simulink model "center_out_3Dv2_ard2"  (Simulink 8.7)
settings: Solver=FixedStepDiscrete  StartTime=0.0  StopTime=Inf  FixedStep=.001  RelTol=1e-3
libraries: slrtlib x6, xpcnilib x5, dspsigops x2, limblab x2, IntelSMIlibR2007b x1, xpcobsoletelib x1, xpcrtudplib x1
CloseFcn:
  | rtwprivate ssgencode ModelCloseRequest rwalk_multi_local_v1
settings Model: Creator=limblab  LastModifiedBy=limblab  ExtModeArmWhenConnect=off
settings SolverCC: EnableConcurrentExecution=on
settings DataIOCC: LimitDataPoints=off  SaveFormat=StructureWithTime  SignalLoggingSaveFormat=ModelDataLogs  SaveState=on  SignalLoggingName=sigsOut
settings OptimizationCC: BlockReduction=off  BooleanDataType=off  OptimizeBlockIOStorage=off  BufferReuse=off  GlobalBufferReuse=off  ExpressionFolding=off  ExpressionDepthLimit=2147483647  LocalBlockOutputs=off  InitFltsAndDblsToZero=on
settings DebuggingCC: SaveWithParameterizedLinksMsg=none  SignalResolutionControl=TryResolveAllWithWarning  MultiTaskDSMMsg=warning  MultiTaskCondExecSysMsg=none  FcnCallInpInsideContextMsg=UseLocalSettings  StateNameClashWarn=warning
settings HardwareCC: ProdIntDivRoundTo=Zero  ProdEndianess=LittleEndian  ProdLongLongMode=on  ProdHWDeviceType=Generic->32-bit x86 compatible  TargetHWDeviceType=32-bit Generic
settings SFSimCC: SimParseCustomCode=off
settings RTWCC: SystemTargetFile=slrt.tlc  TemplateMakefile=slrt_default_tmf  Description=Simulink Real-Time  GenerateReport=on  RTWCompilerOptimization=on
settings SimulinkRealTimeCC: TargetFcnLib=ansi_tfl_tmw.mat  GeneratePreprocessorConditionals=Disable all

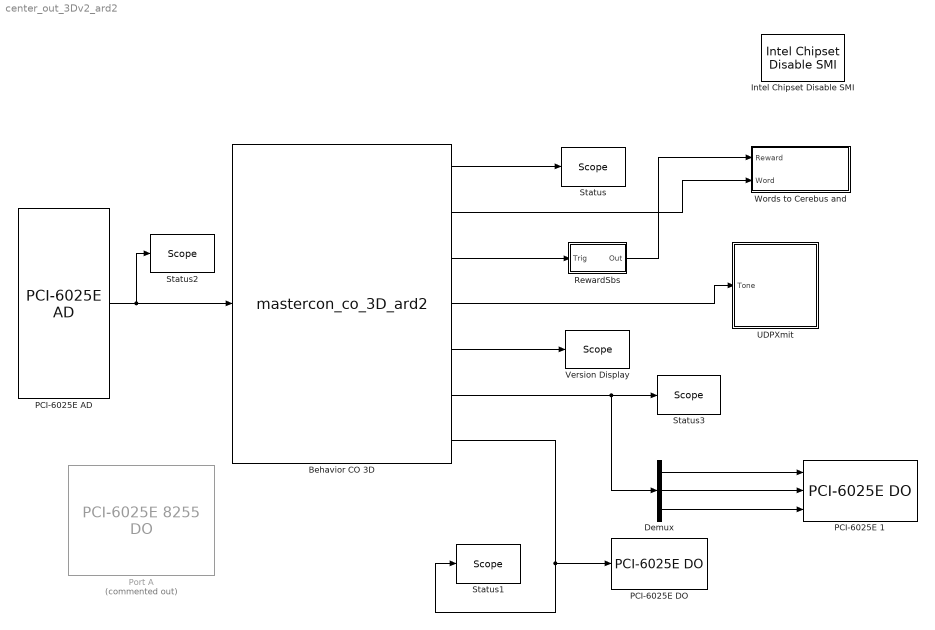
== system center_out_3Dv2_ard2 ==
  Behavior CO 3D : S-Function  FunctionName=mastercon_co_3D_ard2  Parameters=8 10 2.5 1 1 .5 1.5 .75 .25 1 1 10  SFunctionDeploymentMode=off  EnableBusSupport=off
      mask Display:
      | disp('Master Control')
      | port_label('input',1,'Target')
      | port_label('input',2,'Target 2')
      | port_label('output',1,'status')
      | port_label('output',2,'word')
      | port_label('output',3,'reward')
      | port_label('output',4,'tone')
      | port_label('output',5,'version')
      | port_label('output',6,'LEDs')
  Demux : Demux  Outputs=3
  Intel Chipset Disable SMI : IntelSMIlibR2007b/Intel Chipset Disable SMI
  PCI-6025E 1 : xpcnilib/Digital Output/E Series/PCI-6025E DO  channel=[3,7,6]  reset=[0]  initValue=[0]  sampletime=.001  slot=-1
  PCI-6025E AD : xpcnilib/A//D/E Series/PCI-6025E AD  channel=[7]  range=[-10]  coupling=[0]  sampletime=0.001  slot=-1
  PCI-6025E DO : xpcnilib/Digital Output/E Series/PCI-6025E DO  channel=[5]  reset=[1]  initValue=[0]  sampletime=0.001  slot=-1
  Port A : xpcnilib/Digital Output/E Series/PCI-6025E 8255 DO  Commented=on  channel=1:8  port=A  reset=[1]  initValue=[0]  chip=1  sampletime=-1  slot=-1
  RewardSbs : Subsystem
  Status : slrtlib/Displays and Logging/Scope   scopeno=1  scopetype=Target  autostart=on  viewmode=Numerical  formatstr='%6.0f state,%6.0f rewards,%6.0f aborts,%6.0f fails,%6.0f incompl'  grid=on  ylimits=[-10,10]  nosamples=10  noprepostsamples=0  interleave=10  triggermode=FreeRun  triggersignal=1  trigsignalfromport=off  triggerlevel=0.0  triggerslope=Either  triggerscope=1  triggersample=0  filename=data.dat  mode=Lazy  writesize=512  autorestart=off  dynamicfilemode=off  maxwritefilesize=512*1024^2
  Status1 : slrtlib/Displays and Logging/Scope   scopeno=3  scopetype=Target  autostart=on  viewmode=Numerical  formatstr='%1.0f IMU reset'  grid=on  ylimits=[-10,10]  nosamples=10  noprepostsamples=0  interleave=10  triggermode=FreeRun  triggersignal=1  trigsignalfromport=off  triggerlevel=0.0  triggerslope=Either  triggerscope=1  triggersample=0  filename=data.dat  mode=Lazy  writesize=512  autorestart=off  dynamicfilemode=off  maxwritefilesize=512*1024^2
  Status2 : slrtlib/Displays and Logging/Scope   scopeno=4  scopetype=Target  autostart=on  viewmode=Numerical  formatstr='%f Target1'  grid=on  ylimits=[-10,10]  nosamples=10  noprepostsamples=0  interleave=10  triggermode=FreeRun  triggersignal=1  trigsignalfromport=off  triggerlevel=0.0  triggerslope=Either  triggerscope=1  triggersample=0  filename=data.dat  mode=Lazy  writesize=512  autorestart=off  dynamicfilemode=off  maxwritefilesize=512*1024^2
  Status3 : slrtlib/Displays and Logging/Scope   scopeno=5  scopetype=Target  autostart=on  viewmode=Numerical  formatstr='%1.0f Out1,%1.0f Out2,%1.0f Out3'  grid=on  ylimits=[-10,10]  nosamples=10  noprepostsamples=0  interleave=10  triggermode=FreeRun  triggersignal=1  trigsignalfromport=off  triggerlevel=0.0  triggerslope=Either  triggerscope=1  triggersample=0  filename=data.dat  mode=Lazy  writesize=512  autorestart=off  dynamicfilemode=off  maxwritefilesize=512*1024^2
  UDPXmit : Subsystem
  Version Display : slrtlib/Displays and Logging/Scope   scopeno=2  scopetype=Target  autostart=on  viewmode=Numerical  formatstr='%6.0f major,%6.0f minor,%6.0f revision,%6.0f build'  grid=on  ylimits=[-10,10]  nosamples=10  noprepostsamples=0  interleave=10  triggermode=FreeRun  triggersignal=1  trigsignalfromport=off  triggerlevel=0.0  triggerslope=Either  triggerscope=1  triggersample=0  filename=data.dat  mode=Lazy  writesize=512  autorestart=off  dynamicfilemode=off  maxwritefilesize=512*1024^2
  "Words to Cerebus and " : Subsystem
  wires:
  Behavior CO 3D/1 -> Status/1
  Behavior CO 3D/2 -> "Words to Cerebus and "/2(Word)
  Behavior CO 3D/4 -> UDPXmit/1(Tone)
  Behavior CO 3D/5 -> Version Display/1
  Demux/1 -> PCI-6025E 1/1
  Demux/2 -> PCI-6025E 1/2
  Demux/3 -> PCI-6025E 1/3
  Behavior CO 3D/3 -> RewardSbs/1(Trig)
  RewardSbs/1(Out) -> "Words to Cerebus and "/1(Reward)
  Behavior CO 3D/6 -> Demux/1, Status3/1
  PCI-6025E AD/1 -> Behavior CO 3D/1, Status2/1
  Behavior CO 3D/7 -> Status1/1, PCI-6025E DO/1

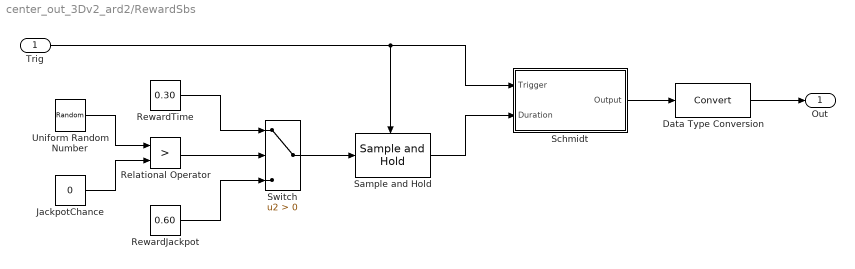
== system center_out_3Dv2_ard2/RewardSbs ==
  Trig : Inport
  Data Type Conversion : DataTypeConversion
  JackpotChance : Constant  Value=0
  Relational Operator : RelationalOperator  Operator=>  OutDataTypeStr=boolean
  RewardJackpot : Constant  Value=0.60
  RewardTime : Constant  Value=0.30
  Sample and Hold : dspsigops/Sample and Hold  trig=Rising edge  initCond=0  latchinput=off
  Schmidt : Subsystem
  Switch : Switch  Criteria=u2 > Threshold  ZeroCross=off
  Uniform Random Number : UniformRandomNumber  Minimum=0  Maximum=100  SampleTime=0.001
  Out : Outport
  wires:
  Trig/1 -> Schmidt/1(Trigger), Sample and Hold/Trigger
  Data Type Conversion/1 -> Out/1
  Schmidt/1(Output) -> Data Type Conversion/1
  Sample and Hold/1 -> Schmidt/2(Duration)
  RewardTime/1 -> Switch/1
  RewardJackpot/1 -> Switch/3
  Switch/1 -> Sample and Hold/1
  Uniform Random Number/1 -> Relational Operator/1
  Relational Operator/1 -> Switch/2
  JackpotChance/1 -> Relational Operator/2

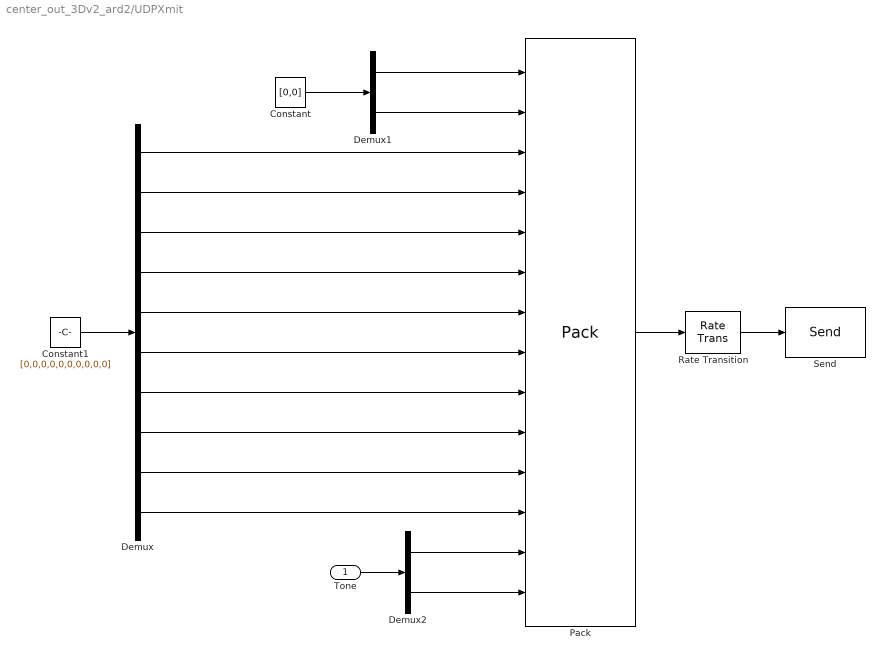
== system center_out_3Dv2_ard2/UDPXmit ==
  Tone : Inport
  Constant : Constant  Value=[0,0]
  Constant1 : Constant  Value=[0,0,0,0,0,0,0,0,0,0]
  Demux : Demux  Outputs=10
  Demux1 : Demux  Outputs=2
  Demux2 : Demux  Outputs=2
  Pack : xpcobsoletelib/Utilities/Pack   datatypes={'double', 'double','double','double','double','double','double','double','double','double','double','double','double','double'}  byteAlign=1
  Rate Transition : RateTransition
  Send : xpcrtudplib/Legacy UDP/Send   ipAddress=192.168.0.2  ipPort=25000  localPort=-1  vblLen=off  sampletime=.02
  wires:
  Rate Transition/1 -> Send/1
  Pack/1 -> Rate Transition/1
  Demux/10 -> Pack/12
  Demux/9 -> Pack/11
  Demux/8 -> Pack/10
  Demux/7 -> Pack/9
  Demux/6 -> Pack/8
  Demux/5 -> Pack/7
  Demux/4 -> Pack/6
  Demux/3 -> Pack/5
  Demux/2 -> Pack/4
  Demux/1 -> Pack/3
  Demux1/1 -> Pack/1
  Demux1/2 -> Pack/2
  Demux2/1 -> Pack/13
  Demux2/2 -> Pack/14
  Tone/1 -> Demux2/1
  Constant1/1 -> Demux/1
  Constant/1 -> Demux1/1

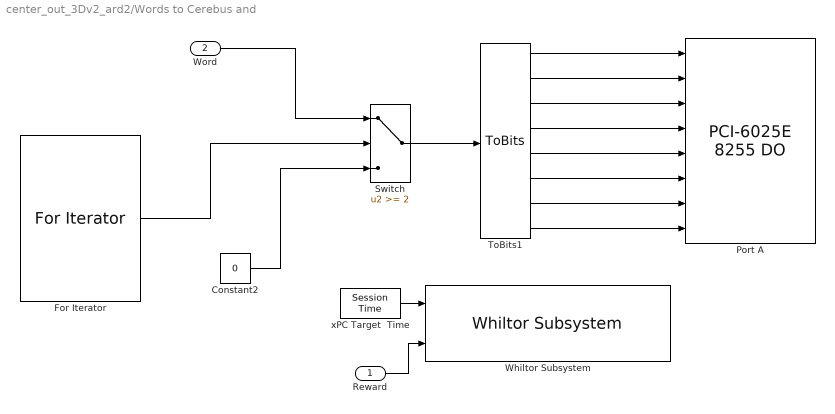
== system center_out_3Dv2_ard2/Words to Cerebus and  ==
  Reward : Inport
  Word : Inport  Port=2
  Constant2 : Constant  Value=0
  For Iterator : ForIterator  IndexMode=Zero-based  IterationVariableDataType=double
  Port A : xpcnilib/Digital Output/E Series/PCI-6025E 8255 DO  channel=1:8  port=A  reset=[1]  initValue=[0]  chip=1  sampletime=-1  slot=-1
  Switch : Switch  Threshold=2
  ToBits1 : limblab/ToBits
  Whiltor Subsystem : limblab/XY Position Subsystem/For Iterator Subsystem/Whiltor Subsystem
      link override "PCI-6025E ": channel=[1,2]
  "xPC Target  Time " : slrtlib/Target Management/Target Information/Session Time   ts=-1
  wires:
  "xPC Target  Time "/1 -> Whiltor Subsystem/1
  Reward/1 -> Whiltor Subsystem/2
  Switch/1 -> ToBits1/1
  Word/1 -> Switch/1
  Constant2/1 -> Switch/3
  ToBits1/8 -> Port A/8
  ToBits1/7 -> Port A/7
  ToBits1/6 -> Port A/6
  ToBits1/5 -> Port A/5
  ToBits1/4 -> Port A/4
  ToBits1/3 -> Port A/3
  ToBits1/2 -> Port A/2
  ToBits1/1 -> Port A/1
  For Iterator/1 -> Switch/2

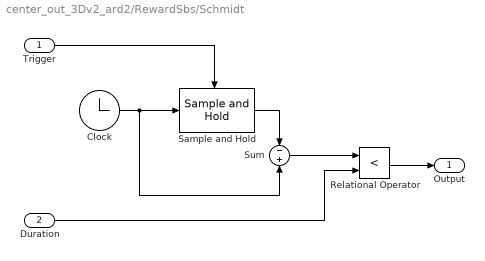
== system center_out_3Dv2_ard2/RewardSbs/Schmidt ==
  Trigger : Inport
  Duration : Inport  Port=2
  Clock : Clock
  Relational Operator : RelationalOperator  Operator=<  OutDataTypeStr=boolean
  Sample and Hold : dspsigops/Sample and Hold  trig=Rising edge  initCond=-1000  latchinput=off
  Sum : Sum  Inputs=-+
  Output : Outport
  wires:
  Clock/1 -> Sum/2, Sample and Hold/1
  Sample and Hold/1 -> Sum/1
  Sum/1 -> Relational Operator/1
  Duration/1 -> Relational Operator/2
  Relational Operator/1 -> Output/1
  Trigger/1 -> Sample and Hold/Trigger
